simulink model "myfirstsimulinkfileb_control101"  (R2023b)
settings: Solver=VariableStepAuto  StartTime=0.0  StopTime=endtime  RelTol=1e-3
undefined symbols (not defined in the file): d, Kp, n
settings Model: Creator=Anthony  LastModifiedBy=Anthony Rossiter
settings DataIOCC: SaveFormat=Array

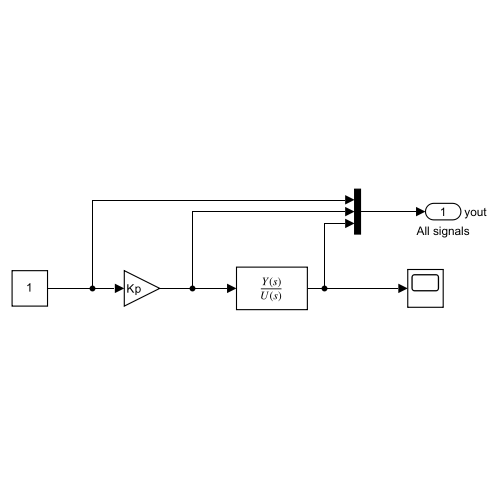
[thumbnail: Simulink's stored preview of the top-level diagram]
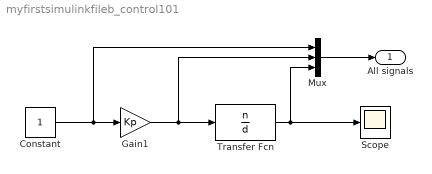
== system myfirstsimulinkfileb_control101 ==
  Constant : Constant
  Gain1 : Gain  Gain=Kp
  Mux : Mux  Inputs=3
  Scope : Scope
  Transfer Fcn : TransferFcn  Numerator=n  Denominator=d
  All signals : Outport  SignalName=yout
  wires:
  Constant/1 -> Mux/1, Gain1/1
  Gain1/1 -> Mux/2, Transfer Fcn/1
  Transfer Fcn/1 -> Mux/3, Scope/1
  Mux/1 -> All signals/1
